simulink model "firefighting_drone_2"  (R2022b)
settings: Solver=FixedStepAuto  StartTime=0.0  StopTime=80  FixedStep=0.1  RelTol=1e-3
(part 2 of 4)

== system firefighting_drone_2/Search for Fire/Seaerch-fire/B4 ==
  In1 : Inport
  Constant : Constant  Value=2
  Demux : Demux  Outputs=3
  Mux : Mux  Inputs=3
  Sum : Sum  Inputs=|++
  O : Outport  VectorParamsAs1DForOutWhenUnconnected=off
  wires:
  Mux/1 -> O/1
  Constant/1 -> Sum/2
  In1/1 -> Demux/1
  Demux/1 -> Mux/1
  Demux/2 -> Sum/1
  Sum/1 -> Mux/2
  Demux/3 -> Mux/3

== system firefighting_drone_2/Search for Fire/Seaerch-fire/B5 ==
  In1 : Inport
  Constant : Constant  Value=18
  Demux : Demux  Outputs=3
  Mux : Mux  Inputs=3
  Sum : Sum  Inputs=|++
  O : Outport  VectorParamsAs1DForOutWhenUnconnected=off
  wires:
  Mux/1 -> O/1
  Demux/3 -> Sum/1
  Constant/1 -> Sum/2
  Sum/1 -> Mux/3
  In1/1 -> Demux/1
  Demux/1 -> Mux/1
  Demux/2 -> Mux/2

== system firefighting_drone_2/Search for Fire/Seaerch-fire/B6 ==
  In1 : Inport
  Constant : Constant  Value=2
  Demux : Demux  Outputs=3
  Mux : Mux  Inputs=3
  Sum : Sum  Inputs=|++
  O : Outport  VectorParamsAs1DForOutWhenUnconnected=off
  wires:
  Mux/1 -> O/1
  Constant/1 -> Sum/2
  In1/1 -> Demux/1
  Demux/1 -> Mux/1
  Demux/2 -> Sum/1
  Sum/1 -> Mux/2
  Demux/3 -> Mux/3

== system firefighting_drone_2/Search for Fire/Seaerch-fire/B7 ==
  In1 : Inport
  Constant : Constant  Value=18
  Demux : Demux  Outputs=3
  Mux : Mux  Inputs=3
  Sum : Sum  Inputs=|+-
  O : Outport  VectorParamsAs1DForOutWhenUnconnected=off
  wires:
  Mux/1 -> O/1
  Demux/3 -> Sum/1
  Constant/1 -> Sum/2
  Sum/1 -> Mux/3
  In1/1 -> Demux/1
  Demux/1 -> Mux/1
  Demux/2 -> Mux/2

== system firefighting_drone_2/Search for Fire/Seaerch-fire/B8 ==
  In1 : Inport
  Constant : Constant  Value=2
  Demux : Demux  Outputs=3
  Mux : Mux  Inputs=3
  Sum : Sum  Inputs=|++
  O : Outport  VectorParamsAs1DForOutWhenUnconnected=off
  wires:
  Mux/1 -> O/1
  Constant/1 -> Sum/2
  In1/1 -> Demux/1
  Demux/1 -> Mux/1
  Demux/2 -> Sum/1
  Sum/1 -> Mux/2
  Demux/3 -> Mux/3

== system firefighting_drone_2/Search for Fire/Seaerch-fire/B9 ==
  In1 : Inport
  Constant : Constant  Value=18
  Demux : Demux  Outputs=3
  Mux : Mux  Inputs=3
  Sum : Sum  Inputs=|++
  O : Outport  VectorParamsAs1DForOutWhenUnconnected=off
  wires:
  Mux/1 -> O/1
  Demux/3 -> Sum/1
  Constant/1 -> Sum/2
  Sum/1 -> Mux/3
  In1/1 -> Demux/1
  Demux/1 -> Mux/1
  Demux/2 -> Mux/2

== system firefighting_drone_2/Search for Fire/Seaerch-fire/Search ==
  Final Coord. : Inport
  Initial Coord. : Inport  Port=2
  Accel : Inport  Port=3
  Constant : Constant
  Constant1 : Constant  Value=0
  Demux : Demux  Outputs=3
  Demux1 : Demux  Outputs=3
  Display : Display
  Display2 : Display
  Move Arm1 : Subsystem
  Move Arm2 : Subsystem
  Move Arm3 : Subsystem
  Mux : Mux  Inputs=3
  Mux1 : Mux  Inputs=3
  Scope : Scope
  Scope1 : Scope  NumInputPorts=3
  Scope2 : Scope
  Scope3 : Scope
  Sum : Sum  Inputs=3
  Switch : Switch  Threshold=3  SaturateOnIntegerOverflow=off  InputSameDT=off
  Flag : Outport  VectorParamsAs1DForOutWhenUnconnected=off
  Current Coord. : Outport  Port=2  VectorParamsAs1DForOutWhenUnconnected=off
  Acc : Outport  Port=3  VectorParamsAs1DForOutWhenUnconnected=off
  wires:
  Demux1/1 -> Mux1/1, Scope3/1, Move Arm1/3(Desired Angle)
  Demux/1 -> Scope2/1, Move Arm1/2(Starting Angle)
  Move Arm3/1(Out1) -> Scope1/3, Mux/3
  Demux/2 -> Move Arm2/2(Starting Angle)
  Accel/1 -> Acc/1, Move Arm2/1(Speed), Move Arm3/1(Speed), Move Arm1/1(Speed)
  Move Arm2/1(Out1) -> Mux/2, Scope1/2
  Move Arm1/1(Out1) -> Mux/1, Scope1/1
  Demux/3 -> Move Arm3/2(Starting Angle)
  Demux1/2 -> Move Arm2/3(Desired Angle), Mux1/2
  Demux1/3 -> Move Arm3/3(Desired Angle), Mux1/3
  Mux/1 -> Display2/1, Current Coord./1, Scope/1
  Mux1/1 -> Display/1
  Initial Coord./1 -> Demux/1
  Final Coord./1 -> Demux1/1
  Move Arm3/2(Done) -> Sum/3
  Move Arm1/2(Done) -> Sum/1
  Move Arm2/2(Done) -> Sum/2
  Constant1/1 -> Switch/3
  Constant/1 -> Switch/1
  Sum/1 -> Switch/2
  Switch/1 -> Flag/1

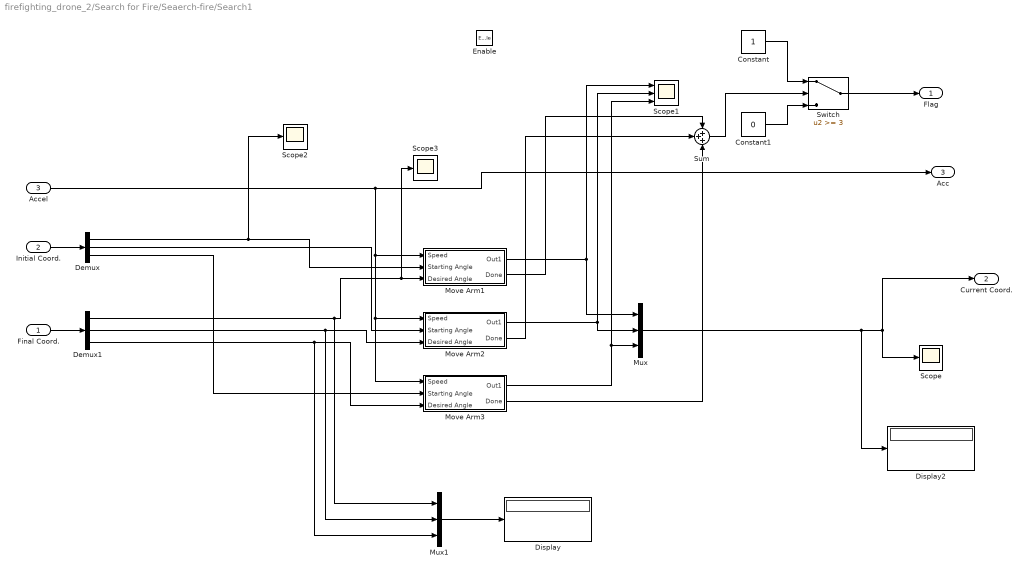
== system firefighting_drone_2/Search for Fire/Seaerch-fire/Search1 ==
  Final Coord. : Inport
  Initial Coord. : Inport  Port=2
  Accel : Inport  Port=3
  Enable : EnablePort
  Constant : Constant
  Constant1 : Constant  Value=0
  Demux : Demux  Outputs=3
  Demux1 : Demux  Outputs=3
  Display : Display
  Display2 : Display
  Move Arm1 : Subsystem
  Move Arm2 : Subsystem
  Move Arm3 : Subsystem
  Mux : Mux  Inputs=3
  Mux1 : Mux  Inputs=3
  Scope : Scope
  Scope1 : Scope  NumInputPorts=3
  Scope2 : Scope
  Scope3 : Scope
  Sum : Sum  Inputs=3
  Switch : Switch  Threshold=3  SaturateOnIntegerOverflow=off  InputSameDT=off
  Flag : Outport  VectorParamsAs1DForOutWhenUnconnected=off
  Current Coord. : Outport  Port=2  VectorParamsAs1DForOutWhenUnconnected=off
  Acc : Outport  Port=3  VectorParamsAs1DForOutWhenUnconnected=off
  wires:
  Demux1/1 -> Mux1/1, Scope3/1, Move Arm1/3(Desired Angle)
  Demux/1 -> Scope2/1, Move Arm1/2(Starting Angle)
  Move Arm3/1(Out1) -> Scope1/3, Mux/3
  Demux/2 -> Move Arm2/2(Starting Angle)
  Accel/1 -> Acc/1, Move Arm2/1(Speed), Move Arm3/1(Speed), Move Arm1/1(Speed)
  Move Arm2/1(Out1) -> Mux/2, Scope1/2
  Move Arm1/1(Out1) -> Mux/1, Scope1/1
  Demux/3 -> Move Arm3/2(Starting Angle)
  Demux1/2 -> Move Arm2/3(Desired Angle), Mux1/2
  Demux1/3 -> Move Arm3/3(Desired Angle), Mux1/3
  Mux/1 -> Display2/1, Current Coord./1, Scope/1
  Mux1/1 -> Display/1
  Initial Coord./1 -> Demux/1
  Final Coord./1 -> Demux1/1
  Move Arm3/2(Done) -> Sum/3
  Move Arm1/2(Done) -> Sum/1
  Move Arm2/2(Done) -> Sum/2
  Constant1/1 -> Switch/3
  Constant/1 -> Switch/1
  Sum/1 -> Switch/2
  Switch/1 -> Flag/1

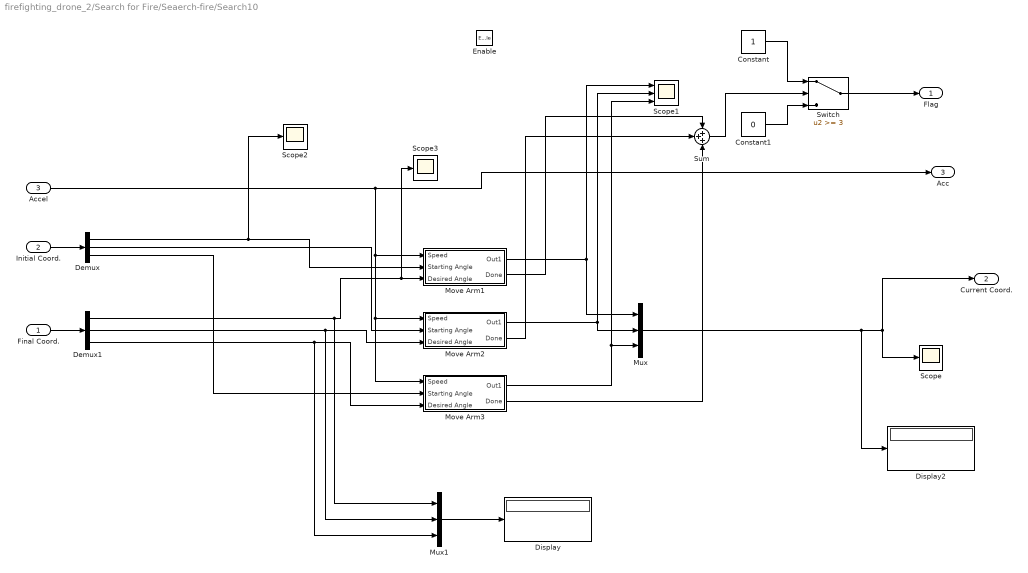
== system firefighting_drone_2/Search for Fire/Seaerch-fire/Search10 ==
  Final Coord. : Inport
  Initial Coord. : Inport  Port=2
  Accel : Inport  Port=3
  Enable : EnablePort
  Constant : Constant
  Constant1 : Constant  Value=0
  Demux : Demux  Outputs=3
  Demux1 : Demux  Outputs=3
  Display : Display
  Display2 : Display
  Move Arm1 : Subsystem
  Move Arm2 : Subsystem
  Move Arm3 : Subsystem
  Mux : Mux  Inputs=3
  Mux1 : Mux  Inputs=3
  Scope : Scope
  Scope1 : Scope  NumInputPorts=3
  Scope2 : Scope
  Scope3 : Scope
  Sum : Sum  Inputs=3
  Switch : Switch  Threshold=3  SaturateOnIntegerOverflow=off  InputSameDT=off
  Flag : Outport  VectorParamsAs1DForOutWhenUnconnected=off
  Current Coord. : Outport  Port=2  VectorParamsAs1DForOutWhenUnconnected=off
  Acc : Outport  Port=3  VectorParamsAs1DForOutWhenUnconnected=off
  wires:
  Demux1/1 -> Mux1/1, Scope3/1, Move Arm1/3(Desired Angle)
  Demux/1 -> Scope2/1, Move Arm1/2(Starting Angle)
  Move Arm3/1(Out1) -> Scope1/3, Mux/3
  Demux/2 -> Move Arm2/2(Starting Angle)
  Accel/1 -> Acc/1, Move Arm2/1(Speed), Move Arm3/1(Speed), Move Arm1/1(Speed)
  Move Arm2/1(Out1) -> Mux/2, Scope1/2
  Move Arm1/1(Out1) -> Mux/1, Scope1/1
  Demux/3 -> Move Arm3/2(Starting Angle)
  Demux1/2 -> Move Arm2/3(Desired Angle), Mux1/2
  Demux1/3 -> Move Arm3/3(Desired Angle), Mux1/3
  Mux/1 -> Display2/1, Current Coord./1, Scope/1
  Mux1/1 -> Display/1
  Initial Coord./1 -> Demux/1
  Final Coord./1 -> Demux1/1
  Move Arm3/2(Done) -> Sum/3
  Move Arm1/2(Done) -> Sum/1
  Move Arm2/2(Done) -> Sum/2
  Constant1/1 -> Switch/3
  Constant/1 -> Switch/1
  Sum/1 -> Switch/2
  Switch/1 -> Flag/1

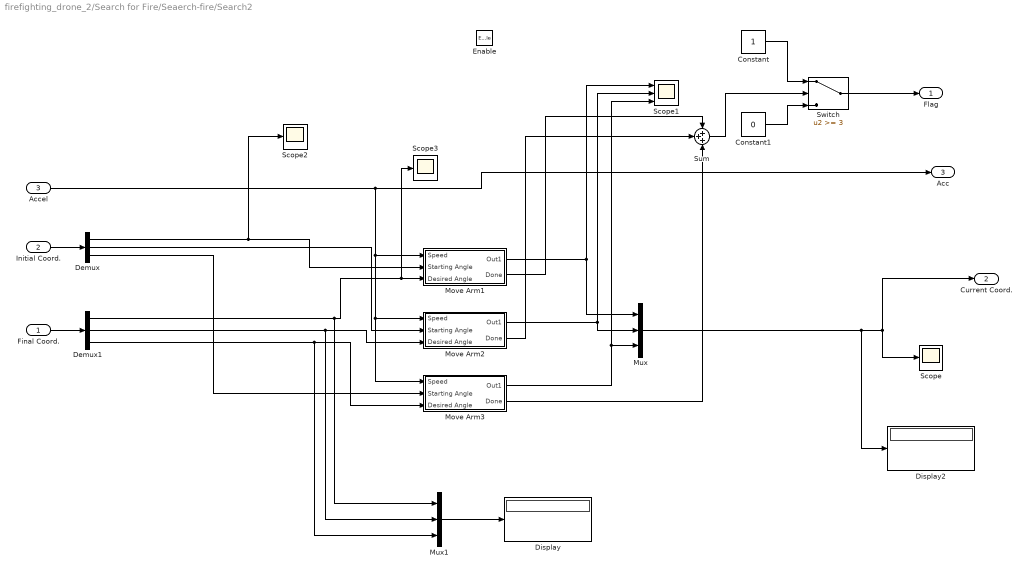
== system firefighting_drone_2/Search for Fire/Seaerch-fire/Search2 ==
  Final Coord. : Inport
  Initial Coord. : Inport  Port=2
  Accel : Inport  Port=3
  Enable : EnablePort
  Constant : Constant
  Constant1 : Constant  Value=0
  Demux : Demux  Outputs=3
  Demux1 : Demux  Outputs=3
  Display : Display
  Display2 : Display
  Move Arm1 : Subsystem
  Move Arm2 : Subsystem
  Move Arm3 : Subsystem
  Mux : Mux  Inputs=3
  Mux1 : Mux  Inputs=3
  Scope : Scope
  Scope1 : Scope  NumInputPorts=3
  Scope2 : Scope
  Scope3 : Scope
  Sum : Sum  Inputs=3
  Switch : Switch  Threshold=3  SaturateOnIntegerOverflow=off  InputSameDT=off
  Flag : Outport  VectorParamsAs1DForOutWhenUnconnected=off
  Current Coord. : Outport  Port=2  VectorParamsAs1DForOutWhenUnconnected=off
  Acc : Outport  Port=3  VectorParamsAs1DForOutWhenUnconnected=off
  wires:
  Demux1/1 -> Mux1/1, Scope3/1, Move Arm1/3(Desired Angle)
  Demux/1 -> Scope2/1, Move Arm1/2(Starting Angle)
  Move Arm3/1(Out1) -> Scope1/3, Mux/3
  Demux/2 -> Move Arm2/2(Starting Angle)
  Accel/1 -> Acc/1, Move Arm2/1(Speed), Move Arm3/1(Speed), Move Arm1/1(Speed)
  Move Arm2/1(Out1) -> Mux/2, Scope1/2
  Move Arm1/1(Out1) -> Mux/1, Scope1/1
  Demux/3 -> Move Arm3/2(Starting Angle)
  Demux1/2 -> Move Arm2/3(Desired Angle), Mux1/2
  Demux1/3 -> Move Arm3/3(Desired Angle), Mux1/3
  Mux/1 -> Display2/1, Current Coord./1, Scope/1
  Mux1/1 -> Display/1
  Initial Coord./1 -> Demux/1
  Final Coord./1 -> Demux1/1
  Move Arm3/2(Done) -> Sum/3
  Move Arm1/2(Done) -> Sum/1
  Move Arm2/2(Done) -> Sum/2
  Constant1/1 -> Switch/3
  Constant/1 -> Switch/1
  Sum/1 -> Switch/2
  Switch/1 -> Flag/1

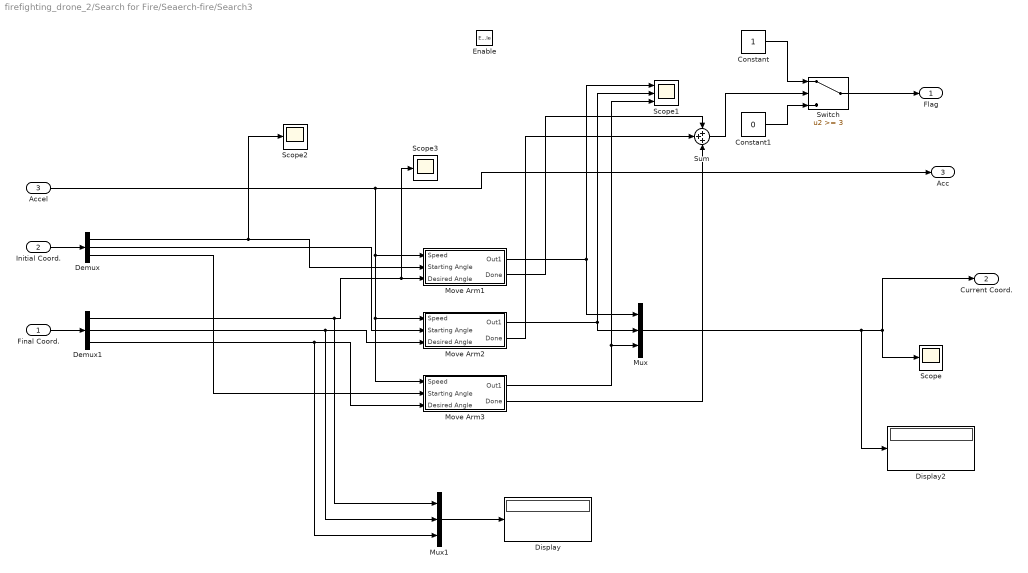
== system firefighting_drone_2/Search for Fire/Seaerch-fire/Search3 ==
  Final Coord. : Inport
  Initial Coord. : Inport  Port=2
  Accel : Inport  Port=3
  Enable : EnablePort
  Constant : Constant
  Constant1 : Constant  Value=0
  Demux : Demux  Outputs=3
  Demux1 : Demux  Outputs=3
  Display : Display
  Display2 : Display
  Move Arm1 : Subsystem
  Move Arm2 : Subsystem
  Move Arm3 : Subsystem
  Mux : Mux  Inputs=3
  Mux1 : Mux  Inputs=3
  Scope : Scope
  Scope1 : Scope  NumInputPorts=3
  Scope2 : Scope
  Scope3 : Scope
  Sum : Sum  Inputs=3
  Switch : Switch  Threshold=3  SaturateOnIntegerOverflow=off  InputSameDT=off
  Flag : Outport  VectorParamsAs1DForOutWhenUnconnected=off
  Current Coord. : Outport  Port=2  VectorParamsAs1DForOutWhenUnconnected=off
  Acc : Outport  Port=3  VectorParamsAs1DForOutWhenUnconnected=off
  wires:
  Demux1/1 -> Mux1/1, Scope3/1, Move Arm1/3(Desired Angle)
  Demux/1 -> Scope2/1, Move Arm1/2(Starting Angle)
  Move Arm3/1(Out1) -> Scope1/3, Mux/3
  Demux/2 -> Move Arm2/2(Starting Angle)
  Accel/1 -> Acc/1, Move Arm2/1(Speed), Move Arm3/1(Speed), Move Arm1/1(Speed)
  Move Arm2/1(Out1) -> Mux/2, Scope1/2
  Move Arm1/1(Out1) -> Mux/1, Scope1/1
  Demux/3 -> Move Arm3/2(Starting Angle)
  Demux1/2 -> Move Arm2/3(Desired Angle), Mux1/2
  Demux1/3 -> Move Arm3/3(Desired Angle), Mux1/3
  Mux/1 -> Display2/1, Current Coord./1, Scope/1
  Mux1/1 -> Display/1
  Initial Coord./1 -> Demux/1
  Final Coord./1 -> Demux1/1
  Move Arm3/2(Done) -> Sum/3
  Move Arm1/2(Done) -> Sum/1
  Move Arm2/2(Done) -> Sum/2
  Constant1/1 -> Switch/3
  Constant/1 -> Switch/1
  Sum/1 -> Switch/2
  Switch/1 -> Flag/1

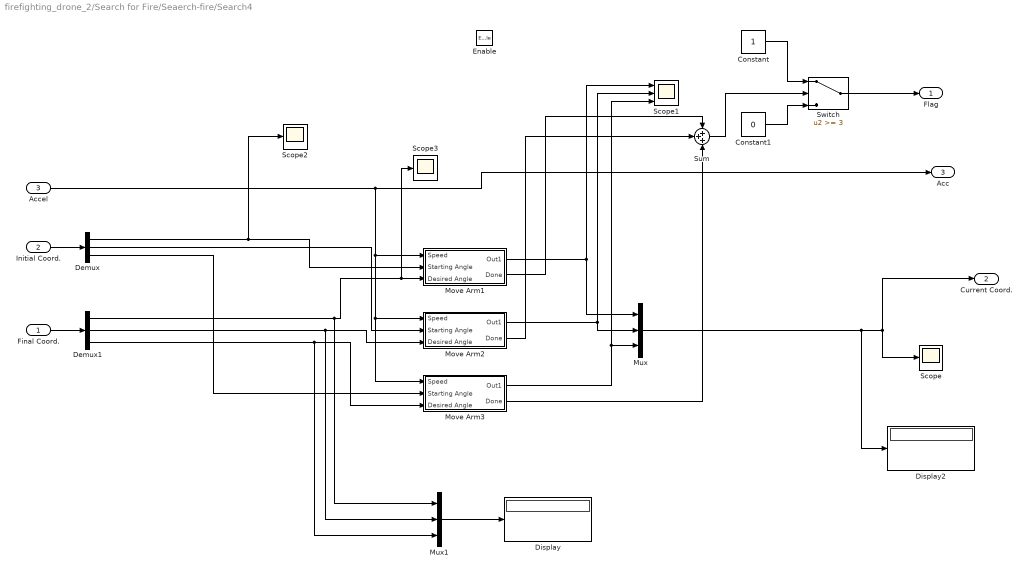
== system firefighting_drone_2/Search for Fire/Seaerch-fire/Search4 ==
  Final Coord. : Inport
  Initial Coord. : Inport  Port=2
  Accel : Inport  Port=3
  Enable : EnablePort
  Constant : Constant
  Constant1 : Constant  Value=0
  Demux : Demux  Outputs=3
  Demux1 : Demux  Outputs=3
  Display : Display
  Display2 : Display
  Move Arm1 : Subsystem
  Move Arm2 : Subsystem
  Move Arm3 : Subsystem
  Mux : Mux  Inputs=3
  Mux1 : Mux  Inputs=3
  Scope : Scope
  Scope1 : Scope  NumInputPorts=3
  Scope2 : Scope
  Scope3 : Scope
  Sum : Sum  Inputs=3
  Switch : Switch  Threshold=3  SaturateOnIntegerOverflow=off  InputSameDT=off
  Flag : Outport  VectorParamsAs1DForOutWhenUnconnected=off
  Current Coord. : Outport  Port=2  VectorParamsAs1DForOutWhenUnconnected=off
  Acc : Outport  Port=3  VectorParamsAs1DForOutWhenUnconnected=off
  wires:
  Demux1/1 -> Mux1/1, Scope3/1, Move Arm1/3(Desired Angle)
  Demux/1 -> Scope2/1, Move Arm1/2(Starting Angle)
  Move Arm3/1(Out1) -> Scope1/3, Mux/3
  Demux/2 -> Move Arm2/2(Starting Angle)
  Accel/1 -> Acc/1, Move Arm2/1(Speed), Move Arm3/1(Speed), Move Arm1/1(Speed)
  Move Arm2/1(Out1) -> Mux/2, Scope1/2
  Move Arm1/1(Out1) -> Mux/1, Scope1/1
  Demux/3 -> Move Arm3/2(Starting Angle)
  Demux1/2 -> Move Arm2/3(Desired Angle), Mux1/2
  Demux1/3 -> Move Arm3/3(Desired Angle), Mux1/3
  Mux/1 -> Display2/1, Current Coord./1, Scope/1
  Mux1/1 -> Display/1
  Initial Coord./1 -> Demux/1
  Final Coord./1 -> Demux1/1
  Move Arm3/2(Done) -> Sum/3
  Move Arm1/2(Done) -> Sum/1
  Move Arm2/2(Done) -> Sum/2
  Constant1/1 -> Switch/3
  Constant/1 -> Switch/1
  Sum/1 -> Switch/2
  Switch/1 -> Flag/1

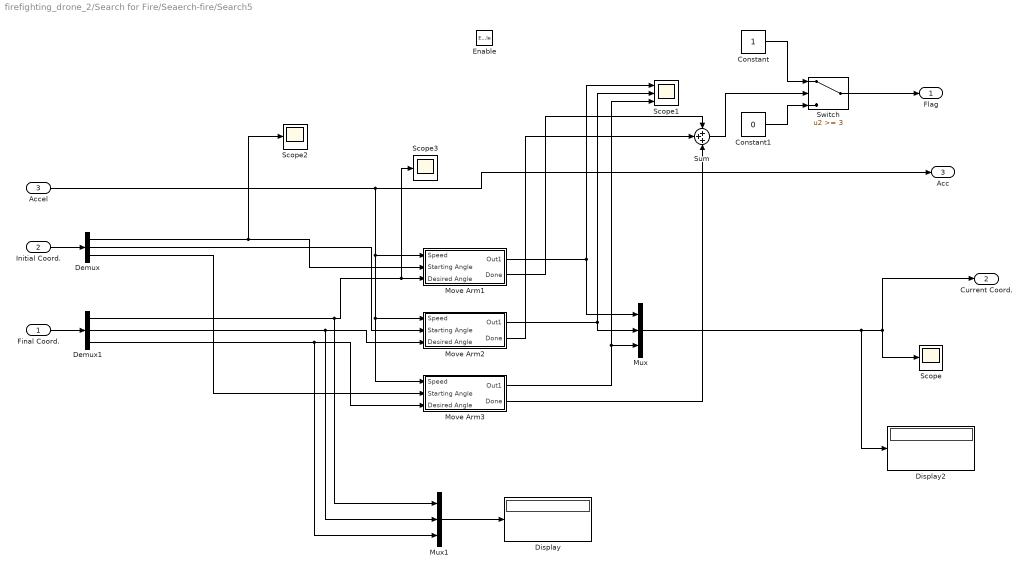
== system firefighting_drone_2/Search for Fire/Seaerch-fire/Search5 ==
  Final Coord. : Inport
  Initial Coord. : Inport  Port=2
  Accel : Inport  Port=3
  Enable : EnablePort
  Constant : Constant
  Constant1 : Constant  Value=0
  Demux : Demux  Outputs=3
  Demux1 : Demux  Outputs=3
  Display : Display
  Display2 : Display
  Move Arm1 : Subsystem
  Move Arm2 : Subsystem
  Move Arm3 : Subsystem
  Mux : Mux  Inputs=3
  Mux1 : Mux  Inputs=3
  Scope : Scope
  Scope1 : Scope  NumInputPorts=3
  Scope2 : Scope
  Scope3 : Scope
  Sum : Sum  Inputs=3
  Switch : Switch  Threshold=3  SaturateOnIntegerOverflow=off  InputSameDT=off
  Flag : Outport  VectorParamsAs1DForOutWhenUnconnected=off
  Current Coord. : Outport  Port=2  VectorParamsAs1DForOutWhenUnconnected=off
  Acc : Outport  Port=3  VectorParamsAs1DForOutWhenUnconnected=off
  wires:
  Demux1/1 -> Mux1/1, Scope3/1, Move Arm1/3(Desired Angle)
  Demux/1 -> Scope2/1, Move Arm1/2(Starting Angle)
  Move Arm3/1(Out1) -> Scope1/3, Mux/3
  Demux/2 -> Move Arm2/2(Starting Angle)
  Accel/1 -> Acc/1, Move Arm2/1(Speed), Move Arm3/1(Speed), Move Arm1/1(Speed)
  Move Arm2/1(Out1) -> Mux/2, Scope1/2
  Move Arm1/1(Out1) -> Mux/1, Scope1/1
  Demux/3 -> Move Arm3/2(Starting Angle)
  Demux1/2 -> Move Arm2/3(Desired Angle), Mux1/2
  Demux1/3 -> Move Arm3/3(Desired Angle), Mux1/3
  Mux/1 -> Display2/1, Current Coord./1, Scope/1
  Mux1/1 -> Display/1
  Initial Coord./1 -> Demux/1
  Final Coord./1 -> Demux1/1
  Move Arm3/2(Done) -> Sum/3
  Move Arm1/2(Done) -> Sum/1
  Move Arm2/2(Done) -> Sum/2
  Constant1/1 -> Switch/3
  Constant/1 -> Switch/1
  Sum/1 -> Switch/2
  Switch/1 -> Flag/1

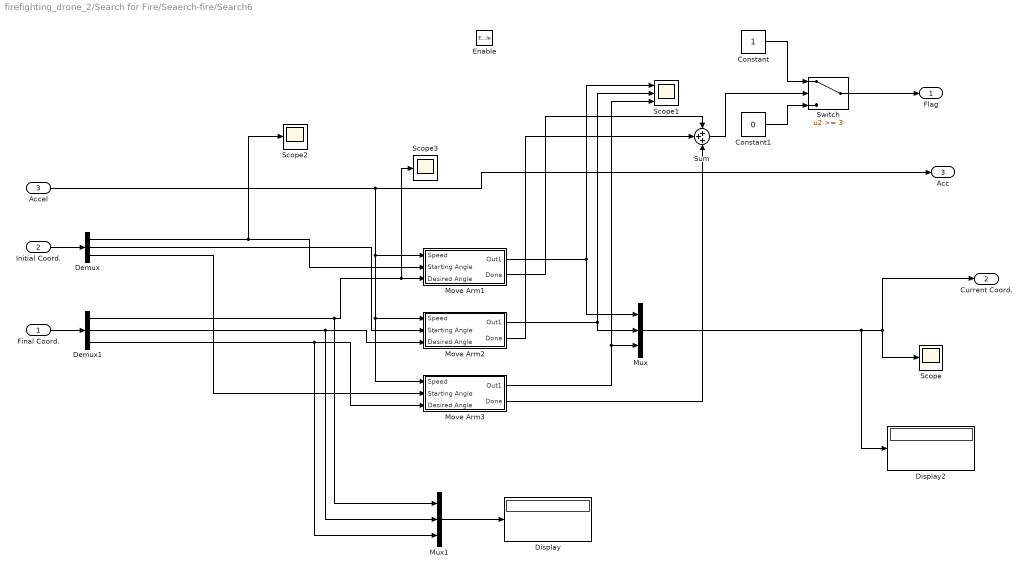
== system firefighting_drone_2/Search for Fire/Seaerch-fire/Search6 ==
  Final Coord. : Inport
  Initial Coord. : Inport  Port=2
  Accel : Inport  Port=3
  Enable : EnablePort
  Constant : Constant
  Constant1 : Constant  Value=0
  Demux : Demux  Outputs=3
  Demux1 : Demux  Outputs=3
  Display : Display
  Display2 : Display
  Move Arm1 : Subsystem
  Move Arm2 : Subsystem
  Move Arm3 : Subsystem
  Mux : Mux  Inputs=3
  Mux1 : Mux  Inputs=3
  Scope : Scope
  Scope1 : Scope  NumInputPorts=3
  Scope2 : Scope
  Scope3 : Scope
  Sum : Sum  Inputs=3
  Switch : Switch  Threshold=3  SaturateOnIntegerOverflow=off  InputSameDT=off
  Flag : Outport  VectorParamsAs1DForOutWhenUnconnected=off
  Current Coord. : Outport  Port=2  VectorParamsAs1DForOutWhenUnconnected=off
  Acc : Outport  Port=3  VectorParamsAs1DForOutWhenUnconnected=off
  wires:
  Demux1/1 -> Mux1/1, Scope3/1, Move Arm1/3(Desired Angle)
  Demux/1 -> Scope2/1, Move Arm1/2(Starting Angle)
  Move Arm3/1(Out1) -> Scope1/3, Mux/3
  Demux/2 -> Move Arm2/2(Starting Angle)
  Accel/1 -> Acc/1, Move Arm2/1(Speed), Move Arm3/1(Speed), Move Arm1/1(Speed)
  Move Arm2/1(Out1) -> Mux/2, Scope1/2
  Move Arm1/1(Out1) -> Mux/1, Scope1/1
  Demux/3 -> Move Arm3/2(Starting Angle)
  Demux1/2 -> Move Arm2/3(Desired Angle), Mux1/2
  Demux1/3 -> Move Arm3/3(Desired Angle), Mux1/3
  Mux/1 -> Display2/1, Current Coord./1, Scope/1
  Mux1/1 -> Display/1
  Initial Coord./1 -> Demux/1
  Final Coord./1 -> Demux1/1
  Move Arm3/2(Done) -> Sum/3
  Move Arm1/2(Done) -> Sum/1
  Move Arm2/2(Done) -> Sum/2
  Constant1/1 -> Switch/3
  Constant/1 -> Switch/1
  Sum/1 -> Switch/2
  Switch/1 -> Flag/1

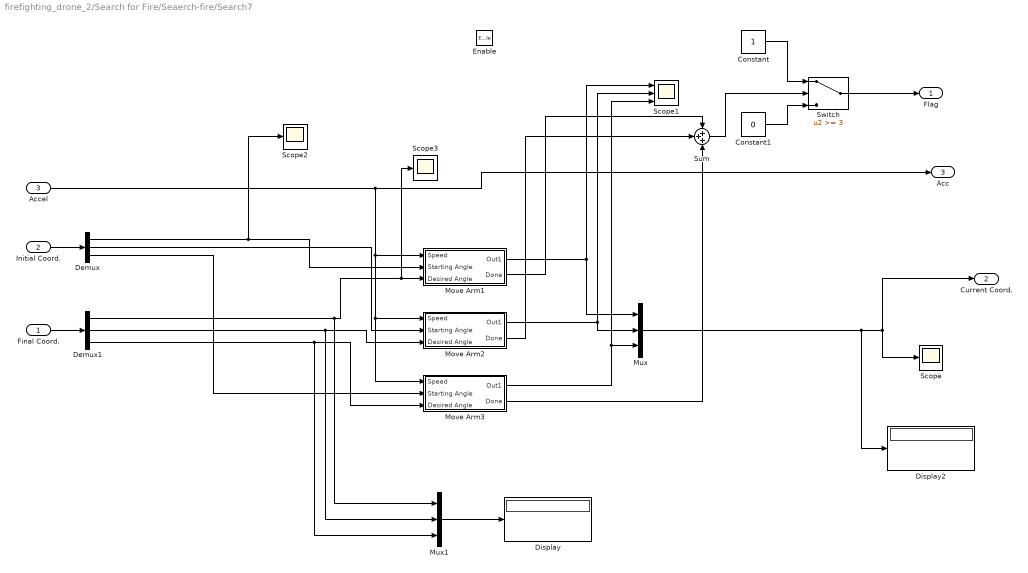
== system firefighting_drone_2/Search for Fire/Seaerch-fire/Search7 ==
  Final Coord. : Inport
  Initial Coord. : Inport  Port=2
  Accel : Inport  Port=3
  Enable : EnablePort
  Constant : Constant
  Constant1 : Constant  Value=0
  Demux : Demux  Outputs=3
  Demux1 : Demux  Outputs=3
  Display : Display
  Display2 : Display
  Move Arm1 : Subsystem
  Move Arm2 : Subsystem
  Move Arm3 : Subsystem
  Mux : Mux  Inputs=3
  Mux1 : Mux  Inputs=3
  Scope : Scope
  Scope1 : Scope  NumInputPorts=3
  Scope2 : Scope
  Scope3 : Scope
  Sum : Sum  Inputs=3
  Switch : Switch  Threshold=3  SaturateOnIntegerOverflow=off  InputSameDT=off
  Flag : Outport  VectorParamsAs1DForOutWhenUnconnected=off
  Current Coord. : Outport  Port=2  VectorParamsAs1DForOutWhenUnconnected=off
  Acc : Outport  Port=3  VectorParamsAs1DForOutWhenUnconnected=off
  wires:
  Demux1/1 -> Mux1/1, Scope3/1, Move Arm1/3(Desired Angle)
  Demux/1 -> Scope2/1, Move Arm1/2(Starting Angle)
  Move Arm3/1(Out1) -> Scope1/3, Mux/3
  Demux/2 -> Move Arm2/2(Starting Angle)
  Accel/1 -> Acc/1, Move Arm2/1(Speed), Move Arm3/1(Speed), Move Arm1/1(Speed)
  Move Arm2/1(Out1) -> Mux/2, Scope1/2
  Move Arm1/1(Out1) -> Mux/1, Scope1/1
  Demux/3 -> Move Arm3/2(Starting Angle)
  Demux1/2 -> Move Arm2/3(Desired Angle), Mux1/2
  Demux1/3 -> Move Arm3/3(Desired Angle), Mux1/3
  Mux/1 -> Display2/1, Current Coord./1, Scope/1
  Mux1/1 -> Display/1
  Initial Coord./1 -> Demux/1
  Final Coord./1 -> Demux1/1
  Move Arm3/2(Done) -> Sum/3
  Move Arm1/2(Done) -> Sum/1
  Move Arm2/2(Done) -> Sum/2
  Constant1/1 -> Switch/3
  Constant/1 -> Switch/1
  Sum/1 -> Switch/2
  Switch/1 -> Flag/1

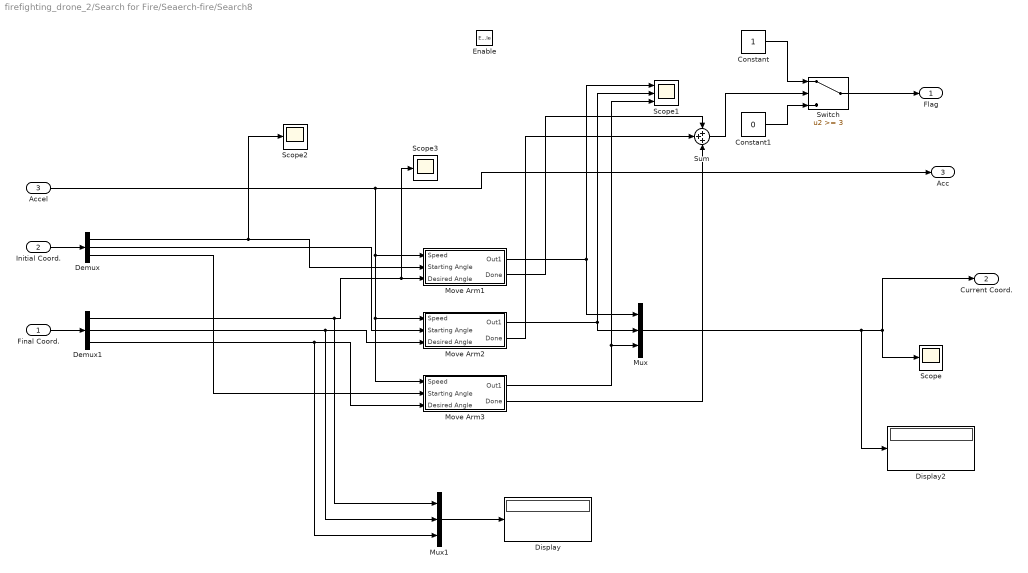
== system firefighting_drone_2/Search for Fire/Seaerch-fire/Search8 ==
  Final Coord. : Inport
  Initial Coord. : Inport  Port=2
  Accel : Inport  Port=3
  Enable : EnablePort
  Constant : Constant
  Constant1 : Constant  Value=0
  Demux : Demux  Outputs=3
  Demux1 : Demux  Outputs=3
  Display : Display
  Display2 : Display
  Move Arm1 : Subsystem
  Move Arm2 : Subsystem
  Move Arm3 : Subsystem
  Mux : Mux  Inputs=3
  Mux1 : Mux  Inputs=3
  Scope : Scope
  Scope1 : Scope  NumInputPorts=3
  Scope2 : Scope
  Scope3 : Scope
  Sum : Sum  Inputs=3
  Switch : Switch  Threshold=3  SaturateOnIntegerOverflow=off  InputSameDT=off
  Flag : Outport  VectorParamsAs1DForOutWhenUnconnected=off
  Current Coord. : Outport  Port=2  VectorParamsAs1DForOutWhenUnconnected=off
  Acc : Outport  Port=3  VectorParamsAs1DForOutWhenUnconnected=off
  wires:
  Demux1/1 -> Mux1/1, Scope3/1, Move Arm1/3(Desired Angle)
  Demux/1 -> Scope2/1, Move Arm1/2(Starting Angle)
  Move Arm3/1(Out1) -> Scope1/3, Mux/3
  Demux/2 -> Move Arm2/2(Starting Angle)
  Accel/1 -> Acc/1, Move Arm2/1(Speed), Move Arm3/1(Speed), Move Arm1/1(Speed)
  Move Arm2/1(Out1) -> Mux/2, Scope1/2
  Move Arm1/1(Out1) -> Mux/1, Scope1/1
  Demux/3 -> Move Arm3/2(Starting Angle)
  Demux1/2 -> Move Arm2/3(Desired Angle), Mux1/2
  Demux1/3 -> Move Arm3/3(Desired Angle), Mux1/3
  Mux/1 -> Display2/1, Current Coord./1, Scope/1
  Mux1/1 -> Display/1
  Initial Coord./1 -> Demux/1
  Final Coord./1 -> Demux1/1
  Move Arm3/2(Done) -> Sum/3
  Move Arm1/2(Done) -> Sum/1
  Move Arm2/2(Done) -> Sum/2
  Constant1/1 -> Switch/3
  Constant/1 -> Switch/1
  Sum/1 -> Switch/2
  Switch/1 -> Flag/1

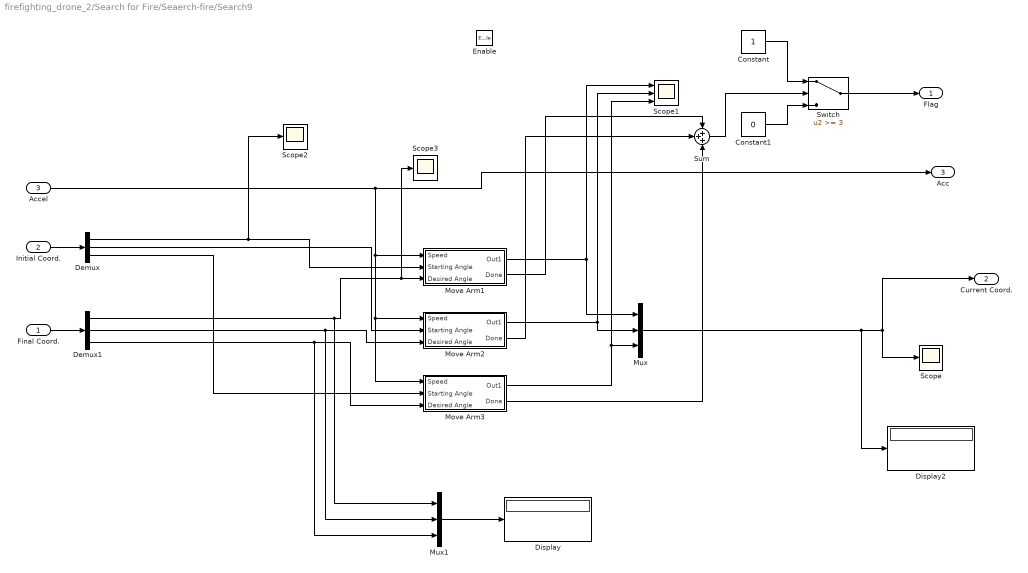
== system firefighting_drone_2/Search for Fire/Seaerch-fire/Search9 ==
  Final Coord. : Inport
  Initial Coord. : Inport  Port=2
  Accel : Inport  Port=3
  Enable : EnablePort
  Constant : Constant
  Constant1 : Constant  Value=0
  Demux : Demux  Outputs=3
  Demux1 : Demux  Outputs=3
  Display : Display
  Display2 : Display
  Move Arm1 : Subsystem
  Move Arm2 : Subsystem
  Move Arm3 : Subsystem
  Mux : Mux  Inputs=3
  Mux1 : Mux  Inputs=3
  Scope : Scope
  Scope1 : Scope  NumInputPorts=3
  Scope2 : Scope
  Scope3 : Scope
  Sum : Sum  Inputs=3
  Switch : Switch  Threshold=3  SaturateOnIntegerOverflow=off  InputSameDT=off
  Flag : Outport  VectorParamsAs1DForOutWhenUnconnected=off
  Current Coord. : Outport  Port=2  VectorParamsAs1DForOutWhenUnconnected=off
  Acc : Outport  Port=3  VectorParamsAs1DForOutWhenUnconnected=off
  wires:
  Demux1/1 -> Mux1/1, Scope3/1, Move Arm1/3(Desired Angle)
  Demux/1 -> Scope2/1, Move Arm1/2(Starting Angle)
  Move Arm3/1(Out1) -> Scope1/3, Mux/3
  Demux/2 -> Move Arm2/2(Starting Angle)
  Accel/1 -> Acc/1, Move Arm2/1(Speed), Move Arm3/1(Speed), Move Arm1/1(Speed)
  Move Arm2/1(Out1) -> Mux/2, Scope1/2
  Move Arm1/1(Out1) -> Mux/1, Scope1/1
  Demux/3 -> Move Arm3/2(Starting Angle)
  Demux1/2 -> Move Arm2/3(Desired Angle), Mux1/2
  Demux1/3 -> Move Arm3/3(Desired Angle), Mux1/3
  Mux/1 -> Display2/1, Current Coord./1, Scope/1
  Mux1/1 -> Display/1
  Initial Coord./1 -> Demux/1
  Final Coord./1 -> Demux1/1
  Move Arm3/2(Done) -> Sum/3
  Move Arm1/2(Done) -> Sum/1
  Move Arm2/2(Done) -> Sum/2
  Constant1/1 -> Switch/3
  Constant/1 -> Switch/1
  Sum/1 -> Switch/2
  Switch/1 -> Flag/1

== system firefighting_drone_2/Search for Fire/Seaerch-fire/Subsystem ==
  "Current " : Inport
  "Desired " : Inport  Port=2
  Abs : Abs  SaturateOnIntegerOverflow=off
  Constant : Constant
  Logical Operator : Logic  Operator=OR  AllPortsSameDT=off  OutDataTypeStr=boolean
  Memory : Memory
  Relational Operator : RelationalOperator  Operator=<=  OutDataTypeStr=boolean  RndMeth=Simplest  InputSameDT=off
  Sum : Sum  Inputs=|+-
  Switch1 : Switch  Criteria=u2 > Threshold  SaturateOnIntegerOverflow=off  InputSameDT=off
  Out1 : Outport  VectorParamsAs1DForOutWhenUnconnected=off
  Done : Outport  Port=2  VectorParamsAs1DForOutWhenUnconnected=off
  wires:
  Switch1/1 -> Out1/1
  "Desired "/1 -> Sum/1, Switch1/1
  "Current "/1 -> Switch1/3, Sum/2
  Sum/1 -> Abs/1
  Abs/1 -> Relational Operator/1
  Constant/1 -> Relational Operator/2
  Relational Operator/1 -> Done/1, Logical Operator/2
  Logical Operator/1 -> Memory/1, Switch1/2
  Memory/1 -> Logical Operator/1

== system firefighting_drone_2/Search for Fire/Seaerch-fire/Subsystem1 ==
  "Current " : Inport
  "Desired " : Inport  Port=2
  Abs : Abs  SaturateOnIntegerOverflow=off
  Constant : Constant
  Logical Operator : Logic  Operator=OR  AllPortsSameDT=off  OutDataTypeStr=boolean
  Memory : Memory
  Relational Operator : RelationalOperator  Operator=<=  OutDataTypeStr=boolean  RndMeth=Simplest  InputSameDT=off
  Sum : Sum  Inputs=|+-
  Switch1 : Switch  Criteria=u2 > Threshold  SaturateOnIntegerOverflow=off  InputSameDT=off
  Out1 : Outport  VectorParamsAs1DForOutWhenUnconnected=off
  Done : Outport  Port=2  VectorParamsAs1DForOutWhenUnconnected=off
  wires:
  Switch1/1 -> Out1/1
  "Desired "/1 -> Sum/1, Switch1/1
  "Current "/1 -> Switch1/3, Sum/2
  Sum/1 -> Abs/1
  Abs/1 -> Relational Operator/1
  Constant/1 -> Relational Operator/2
  Relational Operator/1 -> Done/1, Logical Operator/2
  Logical Operator/1 -> Memory/1, Switch1/2
  Memory/1 -> Logical Operator/1

== system firefighting_drone_2/Search for Fire/Seaerch-fire/Subsystem2 ==
  "Current " : Inport
  "Desired " : Inport  Port=2
  Abs : Abs  SaturateOnIntegerOverflow=off
  Constant : Constant
  Logical Operator : Logic  Operator=OR  AllPortsSameDT=off  OutDataTypeStr=boolean
  Memory : Memory
  Relational Operator : RelationalOperator  Operator=<=  OutDataTypeStr=boolean  RndMeth=Simplest  InputSameDT=off
  Sum : Sum  Inputs=|+-
  Switch1 : Switch  Criteria=u2 > Threshold  SaturateOnIntegerOverflow=off  InputSameDT=off
  Out1 : Outport  VectorParamsAs1DForOutWhenUnconnected=off
  Done : Outport  Port=2  VectorParamsAs1DForOutWhenUnconnected=off
  wires:
  Switch1/1 -> Out1/1
  "Desired "/1 -> Sum/1, Switch1/1
  "Current "/1 -> Switch1/3, Sum/2
  Sum/1 -> Abs/1
  Abs/1 -> Relational Operator/1
  Constant/1 -> Relational Operator/2
  Relational Operator/1 -> Done/1, Logical Operator/2
  Logical Operator/1 -> Memory/1, Switch1/2
  Memory/1 -> Logical Operator/1

== system firefighting_drone_2/Take-off/CoordX/If Action Subsystem ==
  In1 : Inport
  Action Port : ActionPort  ActionPortLabel=if(u1 > 0)
  Out1 : Outport  VectorParamsAs1DForOutWhenUnconnected=off
  wires:
  In1/1 -> Out1/1

== system firefighting_drone_2/Take-off/CoordX/If Action Subsystem1 ==
  In1 : Inport
  Action Port : ActionPort  ActionPortLabel=else
  Out1 : Outport  VectorParamsAs1DForOutWhenUnconnected=off
  wires:
  In1/1 -> Out1/1

== system firefighting_drone_2/Take-off/CoordX/Subsystem ==
  Desired Angle : Inport
  Current Angle : Inport  Port=2
  Abs : Abs  SaturateOnIntegerOverflow=off
  Constant : Constant
  Logical Operator : Logic  Operator=OR  AllPortsSameDT=off  OutDataTypeStr=boolean
  Memory : Memory
  Relational Operator : RelationalOperator  Operator=<=  OutDataTypeStr=boolean  RndMeth=Simplest  InputSameDT=off
  Scope : Scope
  Scope1 : Scope
  Sum : Sum  Inputs=|+-
  Switch1 : Switch  Criteria=u2 > Threshold  SaturateOnIntegerOverflow=off  InputSameDT=off
  Out1 : Outport  VectorParamsAs1DForOutWhenUnconnected=off
  Done : Outport  Port=2  VectorParamsAs1DForOutWhenUnconnected=off
  wires:
  Switch1/1 -> Out1/1
  Desired Angle/1 -> Scope/1, Sum/1, Switch1/1
  Current Angle/1 -> Scope1/1, Switch1/3, Sum/2
  Sum/1 -> Abs/1
  Abs/1 -> Relational Operator/1
  Constant/1 -> Relational Operator/2
  Relational Operator/1 -> Logical Operator/2
  Logical Operator/1 -> Memory/1, Done/1, Switch1/2
  Memory/1 -> Logical Operator/1

== system firefighting_drone_2/Take-off/CoordY/If Action Subsystem ==
  In1 : Inport
  Action Port : ActionPort  ActionPortLabel=if(u1 > 0)
  Out1 : Outport  VectorParamsAs1DForOutWhenUnconnected=off
  wires:
  In1/1 -> Out1/1

== system firefighting_drone_2/Take-off/CoordY/If Action Subsystem1 ==
  In1 : Inport
  Action Port : ActionPort  ActionPortLabel=else
  Out1 : Outport  VectorParamsAs1DForOutWhenUnconnected=off
  wires:
  In1/1 -> Out1/1

== system firefighting_drone_2/Take-off/CoordY/Subsystem ==
  Desired Angle : Inport
  Current Angle : Inport  Port=2
  Abs : Abs  SaturateOnIntegerOverflow=off
  Constant : Constant
  Logical Operator : Logic  Operator=OR  AllPortsSameDT=off  OutDataTypeStr=boolean
  Memory : Memory
  Relational Operator : RelationalOperator  Operator=<=  OutDataTypeStr=boolean  RndMeth=Simplest  InputSameDT=off
  Sum : Sum  Inputs=|+-
  Switch1 : Switch  Criteria=u2 > Threshold  SaturateOnIntegerOverflow=off  InputSameDT=off
  Out1 : Outport  VectorParamsAs1DForOutWhenUnconnected=off
  Done : Outport  Port=2  VectorParamsAs1DForOutWhenUnconnected=off
  wires:
  Switch1/1 -> Out1/1
  Desired Angle/1 -> Sum/1, Switch1/1
  Current Angle/1 -> Switch1/3, Sum/2
  Sum/1 -> Abs/1
  Abs/1 -> Relational Operator/1
  Constant/1 -> Relational Operator/2
  Relational Operator/1 -> Logical Operator/2
  Logical Operator/1 -> Memory/1, Done/1, Switch1/2
  Memory/1 -> Logical Operator/1

== system firefighting_drone_2/Take-off/CoordZ/If Action Subsystem ==
  In1 : Inport
  Action Port : ActionPort  ActionPortLabel=if(u1 > 0)
  Out1 : Outport  VectorParamsAs1DForOutWhenUnconnected=off
  wires:
  In1/1 -> Out1/1

== system firefighting_drone_2/Take-off/CoordZ/If Action Subsystem1 ==
  In1 : Inport
  Action Port : ActionPort  ActionPortLabel=else
  Out1 : Outport  VectorParamsAs1DForOutWhenUnconnected=off
  wires:
  In1/1 -> Out1/1

== system firefighting_drone_2/Take-off/CoordZ/Subsystem ==
  Desired Angle : Inport
  Current Angle : Inport  Port=2
  Abs : Abs  SaturateOnIntegerOverflow=off
  Constant : Constant
  Logical Operator : Logic  Operator=OR  AllPortsSameDT=off  OutDataTypeStr=boolean
  Memory : Memory
  Relational Operator : RelationalOperator  Operator=<=  OutDataTypeStr=boolean  RndMeth=Simplest  InputSameDT=off
  Sum : Sum  Inputs=|+-
  Switch1 : Switch  Criteria=u2 > Threshold  SaturateOnIntegerOverflow=off  InputSameDT=off
  Out1 : Outport  VectorParamsAs1DForOutWhenUnconnected=off
  Done : Outport  Port=2  VectorParamsAs1DForOutWhenUnconnected=off
  wires:
  Switch1/1 -> Out1/1
  Desired Angle/1 -> Sum/1, Switch1/1
  Current Angle/1 -> Switch1/3, Sum/2
  Sum/1 -> Abs/1
  Abs/1 -> Relational Operator/1
  Constant/1 -> Relational Operator/2
  Relational Operator/1 -> Logical Operator/2
  Logical Operator/1 -> Memory/1, Done/1, Switch1/2
  Memory/1 -> Logical Operator/1

== system firefighting_drone_2/Search for Fire/Seaerch-fire/Search/Move Arm1 ==
  Speed : Inport
  Starting Angle : Inport  Port=2
  Desired Angle : Inport  Port=3
  If : If
  If Action Subsystem : Subsystem  TreatAsAtomicUnit=on
  If Action Subsystem1 : Subsystem  TreatAsAtomicUnit=on
  Integrator1 : Integrator
  Scope : Scope
  Scope1 : Scope
  Subsystem : Subsystem
  Sum1 : Sum  Inputs=|++
  Sum2 : Sum  Inputs=|+-
  Sum3 : Sum  Inputs=|-+
  Switch : Switch  Criteria=u2 ~= 0  SaturateOnIntegerOverflow=off  InputSameDT=off
  Out1 : Outport  VectorParamsAs1DForOutWhenUnconnected=off
  Done : Outport  Port=2  VectorParamsAs1DForOutWhenUnconnected=off
  wires:
  Speed/1 -> Integrator1/1
  If Action Subsystem/1(Out1) -> Switch/3
  Sum2/1 -> If/1
  If/2 -> If Action Subsystem1/Action
  Starting Angle/1 -> Sum2/2, Sum3/2, Sum1/2
  Desired Angle/1 -> Scope1/1, Subsystem/1(Desired Angle), Sum2/1
  If Action Subsystem1/1(Out1) -> Switch/1, Switch/2
  If/1 -> If Action Subsystem/Action
  Integrator1/1 -> Sum1/1, Sum3/1
  Sum3/1 -> If Action Subsystem1/1(In1)
  Sum1/1 -> If Action Subsystem/1(In1)
  Switch/1 -> Subsystem/2(Current Angle)
  Subsystem/1(Out1) -> Scope/1, Out1/1
  Subsystem/2(Done) -> Done/1

== system firefighting_drone_2/Search for Fire/Seaerch-fire/Search/Move Arm2 ==
  Speed : Inport
  Starting Angle : Inport  Port=2
  Desired Angle : Inport  Port=3
  If : If
  If Action Subsystem : Subsystem  TreatAsAtomicUnit=on
  If Action Subsystem1 : Subsystem  TreatAsAtomicUnit=on
  Integrator1 : Integrator
  Scope : Scope
  Subsystem : Subsystem
  Sum1 : Sum  Inputs=|++
  Sum2 : Sum  Inputs=|+-
  Sum3 : Sum  Inputs=|-+
  Switch : Switch  Criteria=u2 ~= 0  SaturateOnIntegerOverflow=off  InputSameDT=off
  Out1 : Outport  VectorParamsAs1DForOutWhenUnconnected=off
  Done : Outport  Port=2  VectorParamsAs1DForOutWhenUnconnected=off
  wires:
  Speed/1 -> Integrator1/1
  If Action Subsystem/1(Out1) -> Switch/3
  Sum2/1 -> If/1
  If/2 -> If Action Subsystem1/Action
  Starting Angle/1 -> Sum2/2, Sum3/2, Sum1/2
  Desired Angle/1 -> Subsystem/1(Desired Angle), Sum2/1
  If Action Subsystem1/1(Out1) -> Switch/1, Switch/2
  If/1 -> If Action Subsystem/Action
  Integrator1/1 -> Sum1/1, Sum3/1
  Sum3/1 -> If Action Subsystem1/1(In1)
  Sum1/1 -> If Action Subsystem/1(In1)
  Switch/1 -> Subsystem/2(Current Angle)
  Subsystem/1(Out1) -> Scope/1, Out1/1
  Subsystem/2(Done) -> Done/1

== system firefighting_drone_2/Search for Fire/Seaerch-fire/Search/Move Arm3 ==
  Speed : Inport
  Starting Angle : Inport  Port=2
  Desired Angle : Inport  Port=3
  If : If
  If Action Subsystem : Subsystem  TreatAsAtomicUnit=on
  If Action Subsystem1 : Subsystem  TreatAsAtomicUnit=on
  Integrator1 : Integrator
  Scope : Scope
  Subsystem : Subsystem
  Sum1 : Sum  Inputs=|++
  Sum2 : Sum  Inputs=|+-
  Sum3 : Sum  Inputs=|-+
  Switch : Switch  Criteria=u2 ~= 0  SaturateOnIntegerOverflow=off  InputSameDT=off
  Out1 : Outport  VectorParamsAs1DForOutWhenUnconnected=off
  Done : Outport  Port=2  VectorParamsAs1DForOutWhenUnconnected=off
  wires:
  Speed/1 -> Integrator1/1
  If Action Subsystem/1(Out1) -> Switch/3
  Sum2/1 -> If/1
  If/2 -> If Action Subsystem1/Action
  Starting Angle/1 -> Sum2/2, Sum3/2, Sum1/2
  Desired Angle/1 -> Subsystem/1(Desired Angle), Sum2/1
  If Action Subsystem1/1(Out1) -> Switch/1, Switch/2
  If/1 -> If Action Subsystem/Action
  Integrator1/1 -> Sum1/1, Sum3/1
  Sum3/1 -> If Action Subsystem1/1(In1)
  Sum1/1 -> If Action Subsystem/1(In1)
  Switch/1 -> Subsystem/2(Current Angle)
  Subsystem/1(Out1) -> Scope/1, Out1/1
  Subsystem/2(Done) -> Done/1

== system firefighting_drone_2/Search for Fire/Seaerch-fire/Search1/Move Arm1 ==
  Speed : Inport
  Starting Angle : Inport  Port=2
  Desired Angle : Inport  Port=3
  If : If
  If Action Subsystem : Subsystem  TreatAsAtomicUnit=on
  If Action Subsystem1 : Subsystem  TreatAsAtomicUnit=on
  Integrator1 : Integrator
  Scope : Scope
  Scope1 : Scope
  Subsystem : Subsystem
  Sum1 : Sum  Inputs=|++
  Sum2 : Sum  Inputs=|+-
  Sum3 : Sum  Inputs=|-+
  Switch : Switch  Criteria=u2 ~= 0  SaturateOnIntegerOverflow=off  InputSameDT=off
  Out1 : Outport  VectorParamsAs1DForOutWhenUnconnected=off
  Done : Outport  Port=2  VectorParamsAs1DForOutWhenUnconnected=off
  wires:
  Speed/1 -> Integrator1/1
  If Action Subsystem/1(Out1) -> Switch/3
  Sum2/1 -> If/1
  If/2 -> If Action Subsystem1/Action
  Starting Angle/1 -> Sum2/2, Sum3/2, Sum1/2
  Desired Angle/1 -> Scope1/1, Subsystem/1(Desired Angle), Sum2/1
  If Action Subsystem1/1(Out1) -> Switch/1, Switch/2
  If/1 -> If Action Subsystem/Action
  Integrator1/1 -> Sum1/1, Sum3/1
  Sum3/1 -> If Action Subsystem1/1(In1)
  Sum1/1 -> If Action Subsystem/1(In1)
  Switch/1 -> Subsystem/2(Current Angle)
  Subsystem/1(Out1) -> Scope/1, Out1/1
  Subsystem/2(Done) -> Done/1

== system firefighting_drone_2/Search for Fire/Seaerch-fire/Search1/Move Arm2 ==
  Speed : Inport
  Starting Angle : Inport  Port=2
  Desired Angle : Inport  Port=3
  If : If
  If Action Subsystem : Subsystem  TreatAsAtomicUnit=on
  If Action Subsystem1 : Subsystem  TreatAsAtomicUnit=on
  Integrator1 : Integrator
  Scope : Scope
  Subsystem : Subsystem
  Sum1 : Sum  Inputs=|++
  Sum2 : Sum  Inputs=|+-
  Sum3 : Sum  Inputs=|-+
  Switch : Switch  Criteria=u2 ~= 0  SaturateOnIntegerOverflow=off  InputSameDT=off
  Out1 : Outport  VectorParamsAs1DForOutWhenUnconnected=off
  Done : Outport  Port=2  VectorParamsAs1DForOutWhenUnconnected=off
  wires:
  Speed/1 -> Integrator1/1
  If Action Subsystem/1(Out1) -> Switch/3
  Sum2/1 -> If/1
  If/2 -> If Action Subsystem1/Action
  Starting Angle/1 -> Sum2/2, Sum3/2, Sum1/2
  Desired Angle/1 -> Subsystem/1(Desired Angle), Sum2/1
  If Action Subsystem1/1(Out1) -> Switch/1, Switch/2
  If/1 -> If Action Subsystem/Action
  Integrator1/1 -> Sum1/1, Sum3/1
  Sum3/1 -> If Action Subsystem1/1(In1)
  Sum1/1 -> If Action Subsystem/1(In1)
  Switch/1 -> Subsystem/2(Current Angle)
  Subsystem/1(Out1) -> Scope/1, Out1/1
  Subsystem/2(Done) -> Done/1

== system firefighting_drone_2/Search for Fire/Seaerch-fire/Search1/Move Arm3 ==
  Speed : Inport
  Starting Angle : Inport  Port=2
  Desired Angle : Inport  Port=3
  If : If
  If Action Subsystem : Subsystem  TreatAsAtomicUnit=on
  If Action Subsystem1 : Subsystem  TreatAsAtomicUnit=on
  Integrator1 : Integrator
  Scope : Scope
  Subsystem : Subsystem
  Sum1 : Sum  Inputs=|++
  Sum2 : Sum  Inputs=|+-
  Sum3 : Sum  Inputs=|-+
  Switch : Switch  Criteria=u2 ~= 0  SaturateOnIntegerOverflow=off  InputSameDT=off
  Out1 : Outport  VectorParamsAs1DForOutWhenUnconnected=off
  Done : Outport  Port=2  VectorParamsAs1DForOutWhenUnconnected=off
  wires:
  Speed/1 -> Integrator1/1
  If Action Subsystem/1(Out1) -> Switch/3
  Sum2/1 -> If/1
  If/2 -> If Action Subsystem1/Action
  Starting Angle/1 -> Sum2/2, Sum3/2, Sum1/2
  Desired Angle/1 -> Subsystem/1(Desired Angle), Sum2/1
  If Action Subsystem1/1(Out1) -> Switch/1, Switch/2
  If/1 -> If Action Subsystem/Action
  Integrator1/1 -> Sum1/1, Sum3/1
  Sum3/1 -> If Action Subsystem1/1(In1)
  Sum1/1 -> If Action Subsystem/1(In1)
  Switch/1 -> Subsystem/2(Current Angle)
  Subsystem/1(Out1) -> Scope/1, Out1/1
  Subsystem/2(Done) -> Done/1

== system firefighting_drone_2/Search for Fire/Seaerch-fire/Search10/Move Arm1 ==
  Speed : Inport
  Starting Angle : Inport  Port=2
  Desired Angle : Inport  Port=3
  If : If
  If Action Subsystem : Subsystem  TreatAsAtomicUnit=on
  If Action Subsystem1 : Subsystem  TreatAsAtomicUnit=on
  Integrator1 : Integrator
  Scope : Scope
  Scope1 : Scope
  Subsystem : Subsystem
  Sum1 : Sum  Inputs=|++
  Sum2 : Sum  Inputs=|+-
  Sum3 : Sum  Inputs=|-+
  Switch : Switch  Criteria=u2 ~= 0  SaturateOnIntegerOverflow=off  InputSameDT=off
  Out1 : Outport  VectorParamsAs1DForOutWhenUnconnected=off
  Done : Outport  Port=2  VectorParamsAs1DForOutWhenUnconnected=off
  wires:
  Speed/1 -> Integrator1/1
  If Action Subsystem/1(Out1) -> Switch/3
  Sum2/1 -> If/1
  If/2 -> If Action Subsystem1/Action
  Starting Angle/1 -> Sum2/2, Sum3/2, Sum1/2
  Desired Angle/1 -> Scope1/1, Subsystem/1(Desired Angle), Sum2/1
  If Action Subsystem1/1(Out1) -> Switch/1, Switch/2
  If/1 -> If Action Subsystem/Action
  Integrator1/1 -> Sum1/1, Sum3/1
  Sum3/1 -> If Action Subsystem1/1(In1)
  Sum1/1 -> If Action Subsystem/1(In1)
  Switch/1 -> Subsystem/2(Current Angle)
  Subsystem/1(Out1) -> Scope/1, Out1/1
  Subsystem/2(Done) -> Done/1

== system firefighting_drone_2/Search for Fire/Seaerch-fire/Search10/Move Arm2 ==
  Speed : Inport
  Starting Angle : Inport  Port=2
  Desired Angle : Inport  Port=3
  If : If
  If Action Subsystem : Subsystem  TreatAsAtomicUnit=on
  If Action Subsystem1 : Subsystem  TreatAsAtomicUnit=on
  Integrator1 : Integrator
  Scope : Scope
  Subsystem : Subsystem
  Sum1 : Sum  Inputs=|++
  Sum2 : Sum  Inputs=|+-
  Sum3 : Sum  Inputs=|-+
  Switch : Switch  Criteria=u2 ~= 0  SaturateOnIntegerOverflow=off  InputSameDT=off
  Out1 : Outport  VectorParamsAs1DForOutWhenUnconnected=off
  Done : Outport  Port=2  VectorParamsAs1DForOutWhenUnconnected=off
  wires:
  Speed/1 -> Integrator1/1
  If Action Subsystem/1(Out1) -> Switch/3
  Sum2/1 -> If/1
  If/2 -> If Action Subsystem1/Action
  Starting Angle/1 -> Sum2/2, Sum3/2, Sum1/2
  Desired Angle/1 -> Subsystem/1(Desired Angle), Sum2/1
  If Action Subsystem1/1(Out1) -> Switch/1, Switch/2
  If/1 -> If Action Subsystem/Action
  Integrator1/1 -> Sum1/1, Sum3/1
  Sum3/1 -> If Action Subsystem1/1(In1)
  Sum1/1 -> If Action Subsystem/1(In1)
  Switch/1 -> Subsystem/2(Current Angle)
  Subsystem/1(Out1) -> Scope/1, Out1/1
  Subsystem/2(Done) -> Done/1

== system firefighting_drone_2/Search for Fire/Seaerch-fire/Search10/Move Arm3 ==
  Speed : Inport
  Starting Angle : Inport  Port=2
  Desired Angle : Inport  Port=3
  If : If
  If Action Subsystem : Subsystem  TreatAsAtomicUnit=on
  If Action Subsystem1 : Subsystem  TreatAsAtomicUnit=on
  Integrator1 : Integrator
  Scope : Scope
  Subsystem : Subsystem
  Sum1 : Sum  Inputs=|++
  Sum2 : Sum  Inputs=|+-
  Sum3 : Sum  Inputs=|-+
  Switch : Switch  Criteria=u2 ~= 0  SaturateOnIntegerOverflow=off  InputSameDT=off
  Out1 : Outport  VectorParamsAs1DForOutWhenUnconnected=off
  Done : Outport  Port=2  VectorParamsAs1DForOutWhenUnconnected=off
  wires:
  Speed/1 -> Integrator1/1
  If Action Subsystem/1(Out1) -> Switch/3
  Sum2/1 -> If/1
  If/2 -> If Action Subsystem1/Action
  Starting Angle/1 -> Sum2/2, Sum3/2, Sum1/2
  Desired Angle/1 -> Subsystem/1(Desired Angle), Sum2/1
  If Action Subsystem1/1(Out1) -> Switch/1, Switch/2
  If/1 -> If Action Subsystem/Action
  Integrator1/1 -> Sum1/1, Sum3/1
  Sum3/1 -> If Action Subsystem1/1(In1)
  Sum1/1 -> If Action Subsystem/1(In1)
  Switch/1 -> Subsystem/2(Current Angle)
  Subsystem/1(Out1) -> Scope/1, Out1/1
  Subsystem/2(Done) -> Done/1

== system firefighting_drone_2/Search for Fire/Seaerch-fire/Search2/Move Arm1 ==
  Speed : Inport
  Starting Angle : Inport  Port=2
  Desired Angle : Inport  Port=3
  If : If
  If Action Subsystem : Subsystem  TreatAsAtomicUnit=on
  If Action Subsystem1 : Subsystem  TreatAsAtomicUnit=on
  Integrator1 : Integrator
  Scope : Scope
  Scope1 : Scope
  Subsystem : Subsystem
  Sum1 : Sum  Inputs=|++
  Sum2 : Sum  Inputs=|+-
  Sum3 : Sum  Inputs=|-+
  Switch : Switch  Criteria=u2 ~= 0  SaturateOnIntegerOverflow=off  InputSameDT=off
  Out1 : Outport  VectorParamsAs1DForOutWhenUnconnected=off
  Done : Outport  Port=2  VectorParamsAs1DForOutWhenUnconnected=off
  wires:
  Speed/1 -> Integrator1/1
  If Action Subsystem/1(Out1) -> Switch/3
  Sum2/1 -> If/1
  If/2 -> If Action Subsystem1/Action
  Starting Angle/1 -> Sum2/2, Sum3/2, Sum1/2
  Desired Angle/1 -> Scope1/1, Subsystem/1(Desired Angle), Sum2/1
  If Action Subsystem1/1(Out1) -> Switch/1, Switch/2
  If/1 -> If Action Subsystem/Action
  Integrator1/1 -> Sum1/1, Sum3/1
  Sum3/1 -> If Action Subsystem1/1(In1)
  Sum1/1 -> If Action Subsystem/1(In1)
  Switch/1 -> Subsystem/2(Current Angle)
  Subsystem/1(Out1) -> Scope/1, Out1/1
  Subsystem/2(Done) -> Done/1

== system firefighting_drone_2/Search for Fire/Seaerch-fire/Search2/Move Arm2 ==
  Speed : Inport
  Starting Angle : Inport  Port=2
  Desired Angle : Inport  Port=3
  If : If
  If Action Subsystem : Subsystem  TreatAsAtomicUnit=on
  If Action Subsystem1 : Subsystem  TreatAsAtomicUnit=on
  Integrator1 : Integrator
  Scope : Scope
  Subsystem : Subsystem
  Sum1 : Sum  Inputs=|++
  Sum2 : Sum  Inputs=|+-
  Sum3 : Sum  Inputs=|-+
  Switch : Switch  Criteria=u2 ~= 0  SaturateOnIntegerOverflow=off  InputSameDT=off
  Out1 : Outport  VectorParamsAs1DForOutWhenUnconnected=off
  Done : Outport  Port=2  VectorParamsAs1DForOutWhenUnconnected=off
  wires:
  Speed/1 -> Integrator1/1
  If Action Subsystem/1(Out1) -> Switch/3
  Sum2/1 -> If/1
  If/2 -> If Action Subsystem1/Action
  Starting Angle/1 -> Sum2/2, Sum3/2, Sum1/2
  Desired Angle/1 -> Subsystem/1(Desired Angle), Sum2/1
  If Action Subsystem1/1(Out1) -> Switch/1, Switch/2
  If/1 -> If Action Subsystem/Action
  Integrator1/1 -> Sum1/1, Sum3/1
  Sum3/1 -> If Action Subsystem1/1(In1)
  Sum1/1 -> If Action Subsystem/1(In1)
  Switch/1 -> Subsystem/2(Current Angle)
  Subsystem/1(Out1) -> Scope/1, Out1/1
  Subsystem/2(Done) -> Done/1

== system firefighting_drone_2/Search for Fire/Seaerch-fire/Search2/Move Arm3 ==
  Speed : Inport
  Starting Angle : Inport  Port=2
  Desired Angle : Inport  Port=3
  If : If
  If Action Subsystem : Subsystem  TreatAsAtomicUnit=on
  If Action Subsystem1 : Subsystem  TreatAsAtomicUnit=on
  Integrator1 : Integrator
  Scope : Scope
  Subsystem : Subsystem
  Sum1 : Sum  Inputs=|++
  Sum2 : Sum  Inputs=|+-
  Sum3 : Sum  Inputs=|-+
  Switch : Switch  Criteria=u2 ~= 0  SaturateOnIntegerOverflow=off  InputSameDT=off
  Out1 : Outport  VectorParamsAs1DForOutWhenUnconnected=off
  Done : Outport  Port=2  VectorParamsAs1DForOutWhenUnconnected=off
  wires:
  Speed/1 -> Integrator1/1
  If Action Subsystem/1(Out1) -> Switch/3
  Sum2/1 -> If/1
  If/2 -> If Action Subsystem1/Action
  Starting Angle/1 -> Sum2/2, Sum3/2, Sum1/2
  Desired Angle/1 -> Subsystem/1(Desired Angle), Sum2/1
  If Action Subsystem1/1(Out1) -> Switch/1, Switch/2
  If/1 -> If Action Subsystem/Action
  Integrator1/1 -> Sum1/1, Sum3/1
  Sum3/1 -> If Action Subsystem1/1(In1)
  Sum1/1 -> If Action Subsystem/1(In1)
  Switch/1 -> Subsystem/2(Current Angle)
  Subsystem/1(Out1) -> Scope/1, Out1/1
  Subsystem/2(Done) -> Done/1

== system firefighting_drone_2/Search for Fire/Seaerch-fire/Search3/Move Arm1 ==
  Speed : Inport
  Starting Angle : Inport  Port=2
  Desired Angle : Inport  Port=3
  If : If
  If Action Subsystem : Subsystem  TreatAsAtomicUnit=on
  If Action Subsystem1 : Subsystem  TreatAsAtomicUnit=on
  Integrator1 : Integrator
  Scope : Scope
  Scope1 : Scope
  Subsystem : Subsystem
  Sum1 : Sum  Inputs=|++
  Sum2 : Sum  Inputs=|+-
  Sum3 : Sum  Inputs=|-+
  Switch : Switch  Criteria=u2 ~= 0  SaturateOnIntegerOverflow=off  InputSameDT=off
  Out1 : Outport  VectorParamsAs1DForOutWhenUnconnected=off
  Done : Outport  Port=2  VectorParamsAs1DForOutWhenUnconnected=off
  wires:
  Speed/1 -> Integrator1/1
  If Action Subsystem/1(Out1) -> Switch/3
  Sum2/1 -> If/1
  If/2 -> If Action Subsystem1/Action
  Starting Angle/1 -> Sum2/2, Sum3/2, Sum1/2
  Desired Angle/1 -> Scope1/1, Subsystem/1(Desired Angle), Sum2/1
  If Action Subsystem1/1(Out1) -> Switch/1, Switch/2
  If/1 -> If Action Subsystem/Action
  Integrator1/1 -> Sum1/1, Sum3/1
  Sum3/1 -> If Action Subsystem1/1(In1)
  Sum1/1 -> If Action Subsystem/1(In1)
  Switch/1 -> Subsystem/2(Current Angle)
  Subsystem/1(Out1) -> Scope/1, Out1/1
  Subsystem/2(Done) -> Done/1

== system firefighting_drone_2/Search for Fire/Seaerch-fire/Search3/Move Arm2 ==
  Speed : Inport
  Starting Angle : Inport  Port=2
  Desired Angle : Inport  Port=3
  If : If
  If Action Subsystem : Subsystem  TreatAsAtomicUnit=on
  If Action Subsystem1 : Subsystem  TreatAsAtomicUnit=on
  Integrator1 : Integrator
  Scope : Scope
  Subsystem : Subsystem
  Sum1 : Sum  Inputs=|++
  Sum2 : Sum  Inputs=|+-
  Sum3 : Sum  Inputs=|-+
  Switch : Switch  Criteria=u2 ~= 0  SaturateOnIntegerOverflow=off  InputSameDT=off
  Out1 : Outport  VectorParamsAs1DForOutWhenUnconnected=off
  Done : Outport  Port=2  VectorParamsAs1DForOutWhenUnconnected=off
  wires:
  Speed/1 -> Integrator1/1
  If Action Subsystem/1(Out1) -> Switch/3
  Sum2/1 -> If/1
  If/2 -> If Action Subsystem1/Action
  Starting Angle/1 -> Sum2/2, Sum3/2, Sum1/2
  Desired Angle/1 -> Subsystem/1(Desired Angle), Sum2/1
  If Action Subsystem1/1(Out1) -> Switch/1, Switch/2
  If/1 -> If Action Subsystem/Action
  Integrator1/1 -> Sum1/1, Sum3/1
  Sum3/1 -> If Action Subsystem1/1(In1)
  Sum1/1 -> If Action Subsystem/1(In1)
  Switch/1 -> Subsystem/2(Current Angle)
  Subsystem/1(Out1) -> Scope/1, Out1/1
  Subsystem/2(Done) -> Done/1

== system firefighting_drone_2/Search for Fire/Seaerch-fire/Search3/Move Arm3 ==
  Speed : Inport
  Starting Angle : Inport  Port=2
  Desired Angle : Inport  Port=3
  If : If
  If Action Subsystem : Subsystem  TreatAsAtomicUnit=on
  If Action Subsystem1 : Subsystem  TreatAsAtomicUnit=on
  Integrator1 : Integrator
  Scope : Scope
  Subsystem : Subsystem
  Sum1 : Sum  Inputs=|++
  Sum2 : Sum  Inputs=|+-
  Sum3 : Sum  Inputs=|-+
  Switch : Switch  Criteria=u2 ~= 0  SaturateOnIntegerOverflow=off  InputSameDT=off
  Out1 : Outport  VectorParamsAs1DForOutWhenUnconnected=off
  Done : Outport  Port=2  VectorParamsAs1DForOutWhenUnconnected=off
  wires:
  Speed/1 -> Integrator1/1
  If Action Subsystem/1(Out1) -> Switch/3
  Sum2/1 -> If/1
  If/2 -> If Action Subsystem1/Action
  Starting Angle/1 -> Sum2/2, Sum3/2, Sum1/2
  Desired Angle/1 -> Subsystem/1(Desired Angle), Sum2/1
  If Action Subsystem1/1(Out1) -> Switch/1, Switch/2
  If/1 -> If Action Subsystem/Action
  Integrator1/1 -> Sum1/1, Sum3/1
  Sum3/1 -> If Action Subsystem1/1(In1)
  Sum1/1 -> If Action Subsystem/1(In1)
  Switch/1 -> Subsystem/2(Current Angle)
  Subsystem/1(Out1) -> Scope/1, Out1/1
  Subsystem/2(Done) -> Done/1

== system firefighting_drone_2/Search for Fire/Seaerch-fire/Search4/Move Arm1 ==
  Speed : Inport
  Starting Angle : Inport  Port=2
  Desired Angle : Inport  Port=3
  If : If
  If Action Subsystem : Subsystem  TreatAsAtomicUnit=on
  If Action Subsystem1 : Subsystem  TreatAsAtomicUnit=on
  Integrator1 : Integrator
  Scope : Scope
  Scope1 : Scope
  Subsystem : Subsystem
  Sum1 : Sum  Inputs=|++
  Sum2 : Sum  Inputs=|+-
  Sum3 : Sum  Inputs=|-+
  Switch : Switch  Criteria=u2 ~= 0  SaturateOnIntegerOverflow=off  InputSameDT=off
  Out1 : Outport  VectorParamsAs1DForOutWhenUnconnected=off
  Done : Outport  Port=2  VectorParamsAs1DForOutWhenUnconnected=off
  wires:
  Speed/1 -> Integrator1/1
  If Action Subsystem/1(Out1) -> Switch/3
  Sum2/1 -> If/1
  If/2 -> If Action Subsystem1/Action
  Starting Angle/1 -> Sum2/2, Sum3/2, Sum1/2
  Desired Angle/1 -> Scope1/1, Subsystem/1(Desired Angle), Sum2/1
  If Action Subsystem1/1(Out1) -> Switch/1, Switch/2
  If/1 -> If Action Subsystem/Action
  Integrator1/1 -> Sum1/1, Sum3/1
  Sum3/1 -> If Action Subsystem1/1(In1)
  Sum1/1 -> If Action Subsystem/1(In1)
  Switch/1 -> Subsystem/2(Current Angle)
  Subsystem/1(Out1) -> Scope/1, Out1/1
  Subsystem/2(Done) -> Done/1

== system firefighting_drone_2/Search for Fire/Seaerch-fire/Search4/Move Arm2 ==
  Speed : Inport
  Starting Angle : Inport  Port=2
  Desired Angle : Inport  Port=3
  If : If
  If Action Subsystem : Subsystem  TreatAsAtomicUnit=on
  If Action Subsystem1 : Subsystem  TreatAsAtomicUnit=on
  Integrator1 : Integrator
  Scope : Scope
  Subsystem : Subsystem
  Sum1 : Sum  Inputs=|++
  Sum2 : Sum  Inputs=|+-
  Sum3 : Sum  Inputs=|-+
  Switch : Switch  Criteria=u2 ~= 0  SaturateOnIntegerOverflow=off  InputSameDT=off
  Out1 : Outport  VectorParamsAs1DForOutWhenUnconnected=off
  Done : Outport  Port=2  VectorParamsAs1DForOutWhenUnconnected=off
  wires:
  Speed/1 -> Integrator1/1
  If Action Subsystem/1(Out1) -> Switch/3
  Sum2/1 -> If/1
  If/2 -> If Action Subsystem1/Action
  Starting Angle/1 -> Sum2/2, Sum3/2, Sum1/2
  Desired Angle/1 -> Subsystem/1(Desired Angle), Sum2/1
  If Action Subsystem1/1(Out1) -> Switch/1, Switch/2
  If/1 -> If Action Subsystem/Action
  Integrator1/1 -> Sum1/1, Sum3/1
  Sum3/1 -> If Action Subsystem1/1(In1)
  Sum1/1 -> If Action Subsystem/1(In1)
  Switch/1 -> Subsystem/2(Current Angle)
  Subsystem/1(Out1) -> Scope/1, Out1/1
  Subsystem/2(Done) -> Done/1

== system firefighting_drone_2/Search for Fire/Seaerch-fire/Search4/Move Arm3 ==
  Speed : Inport
  Starting Angle : Inport  Port=2
  Desired Angle : Inport  Port=3
  If : If
  If Action Subsystem : Subsystem  TreatAsAtomicUnit=on
  If Action Subsystem1 : Subsystem  TreatAsAtomicUnit=on
  Integrator1 : Integrator
  Scope : Scope
  Subsystem : Subsystem
  Sum1 : Sum  Inputs=|++
  Sum2 : Sum  Inputs=|+-
  Sum3 : Sum  Inputs=|-+
  Switch : Switch  Criteria=u2 ~= 0  SaturateOnIntegerOverflow=off  InputSameDT=off
  Out1 : Outport  VectorParamsAs1DForOutWhenUnconnected=off
  Done : Outport  Port=2  VectorParamsAs1DForOutWhenUnconnected=off
  wires:
  Speed/1 -> Integrator1/1
  If Action Subsystem/1(Out1) -> Switch/3
  Sum2/1 -> If/1
  If/2 -> If Action Subsystem1/Action
  Starting Angle/1 -> Sum2/2, Sum3/2, Sum1/2
  Desired Angle/1 -> Subsystem/1(Desired Angle), Sum2/1
  If Action Subsystem1/1(Out1) -> Switch/1, Switch/2
  If/1 -> If Action Subsystem/Action
  Integrator1/1 -> Sum1/1, Sum3/1
  Sum3/1 -> If Action Subsystem1/1(In1)
  Sum1/1 -> If Action Subsystem/1(In1)
  Switch/1 -> Subsystem/2(Current Angle)
  Subsystem/1(Out1) -> Scope/1, Out1/1
  Subsystem/2(Done) -> Done/1
